simulink model "Moter_Sensor_Integral"  (R2021a)
settings: Solver=FixedStepDiscrete  StartTime=0.0  StopTime=Inf  FixedStep=0.05  RelTol=1e-3
undefined symbols (not defined in the file or in its folder): DiscIntNeverNeededParam
libraries: arduinolib x4, arduinosensorlib x1
settings Model: SimulationMode=external  SILPILModeSetting=veronly  ExtModeTrigDuration=2  Creator=Samsung  LastModifiedBy=Samsung
settings SolverCC: AutoInsertRateTranBlk=on
settings OptimizationCC: EnhancedBackFolding=on  PassReuseOutputArgsAs=Individual arguments  ZeroExternalMemoryAtStartup=off  ZeroInternalMemoryAtStartup=off  MaxStackSize=64  OptimizeBlockOrder=speed  DifferentSizesBufferReuse=on  OptimizationCustomize=off  EfficientTunableParamExpr=on
settings DebuggingCC: ParameterTunabilityLossMsg=error
settings HardwareCC: ProdBitPerPointer=32  ProdBitPerSizeT=32  ProdBitPerPtrDiffT=32  ProdLargestAtomicInteger=Long  ProdLargestAtomicFloat=Double  ProdWordSize=32  ProdHWDeviceType=ARM Compatible->ARM Cortex
settings SFSimCC: MATLABDynamicMemAlloc=off
settings RTWCC: SystemTargetFile=ert.tlc  HardwareBoard=Arduino Nano 33 BLE Sense  TemplateMakefile=ert_default_tmf  Toolchain=Arduino ARM MBED  BuildConfiguration=Faster Runs
settings CodeAppCC: ForceParamTrailComments=on  IgnoreCustomStorageClasses=off  OperatorAnnotations=on  SimulinkDataObjDesc=on  SFDataObjDesc=on  InsertBlockDesc=on
settings ERTTargetCC: SupportContinuousTime=on  SupportVariableSizeSignals=on  ExtMode=on  ExtModeTransport=3  ExtModeStaticAlloc=on  ExtModeStaticAllocSize=65536  ExtModeMexFile=ext_xcp  ExtModeMexArgs=0 16 921600  ExtModeIntrfLevel=Level2 - Open

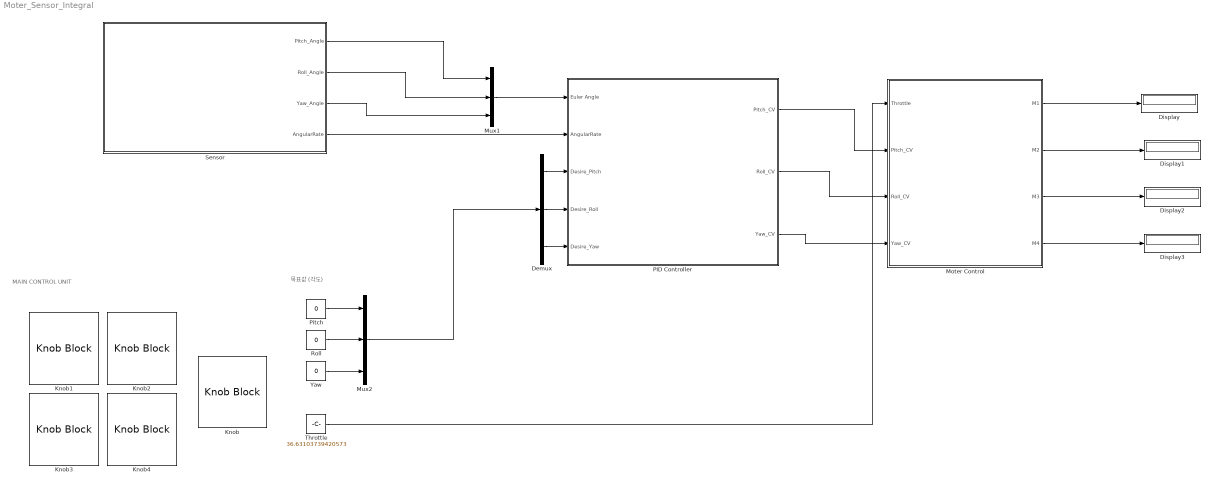
== system Moter_Sensor_Integral ==
  note: MAIN CONTROL UNIT
  note: 목표값 (각도)
  Demux : Demux  Outputs=3
  Display{,1..3} (4 alike) : Display
  Knob : KnobBlock  ScaleMax=200
  Knob1 : KnobBlock  ScaleMax=15
  Knob2 : KnobBlock  ScaleMax=0.1
  Knob3 : KnobBlock  ScaleMin=1  ScaleMax=15
  Knob4 : KnobBlock  ScaleMax=0.1
  Moter Control : Subsystem
  Mux1 : Mux  Inputs=3
  Mux2 : Mux  Inputs=3
  PID Controller : Subsystem
  Pitch : Constant  Value=0
  Roll : Constant  Value=0
  Sensor : Subsystem
  Throttle : Constant  Value=36.63103739420573
  Yaw : Constant  Value=0
  wires:
  PID Controller/1(Pitch_CV) -> Moter Control/2(Pitch_CV)
  PID Controller/2(Roll_CV) -> Moter Control/3(Roll_CV)
  PID Controller/3(Yaw_CV) -> Moter Control/4(Yaw_CV)
  Mux1/1 -> PID Controller/1(Euler Angle)
  Sensor/1(" Pitch_Angle") -> Mux1/1
  Sensor/2(" Roll_Angle") -> Mux1/2
  Sensor/3(Yaw_Angle) -> Mux1/3
  Roll/1 -> Mux2/2
  Pitch/1 -> Mux2/1
  Yaw/1 -> Mux2/3
  Sensor/4(AngularRate) -> PID Controller/2(AngularRate)
  Demux/2 -> PID Controller/4(Desire_Roll)
  Demux/1 -> PID Controller/3(Desire_Pitch)
  Demux/3 -> PID Controller/5(Desire_Yaw)
  Mux2/1 -> Demux/1
  Throttle/1 -> Moter Control/1(Throttle)
  Moter Control/4(M4) -> Display3/1
  Moter Control/3(M3) -> Display2/1
  Moter Control/2(M2) -> Display1/1
  Moter Control/1(M1) -> Display/1

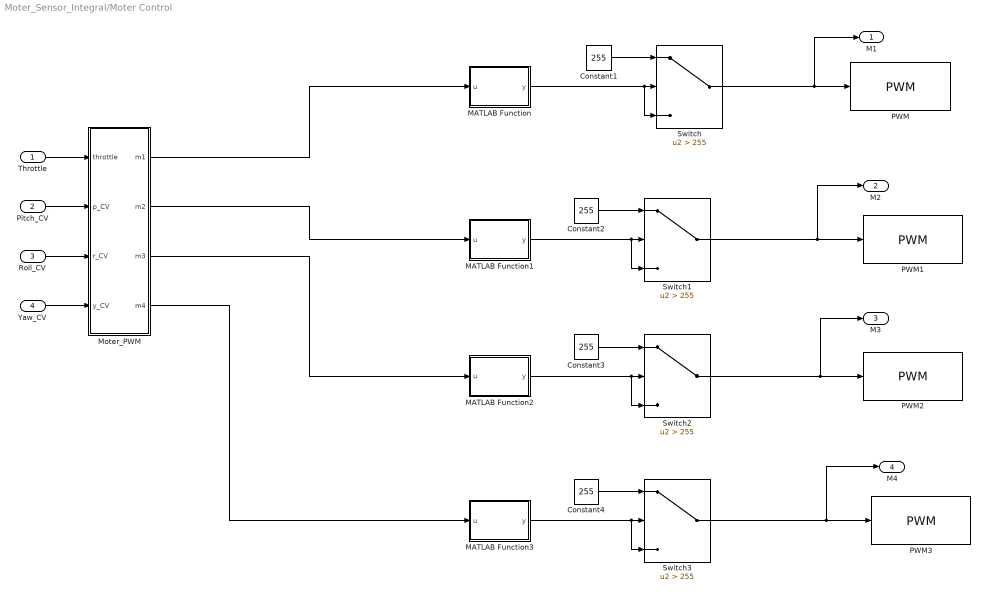
== system Moter_Sensor_Integral/Moter Control ==
  Throttle : Inport
  Pitch_CV : Inport  Port=2
  Roll_CV : Inport  Port=3
  Yaw_CV : Inport  Port=4
  Constant{1..4} (4 alike) : Constant  Value=255
  MATLAB Function : MATLAB Function  TreatAsAtomicUnit=on
  MATLAB Function1 : MATLAB Function  TreatAsAtomicUnit=on
  MATLAB Function2 : MATLAB Function  TreatAsAtomicUnit=on
  MATLAB Function3 : MATLAB Function  TreatAsAtomicUnit=on
  Moter_PWM : MATLAB Function  TreatAsAtomicUnit=on
  PWM : arduinolib/PWM  pinNumber=12  frequencyType=Default  desiredFrequency=490.2  achievableFrequency=490.2
  PWM1 : arduinolib/PWM  pinNumber=8  frequencyType=Default  desiredFrequency=490.2  achievableFrequency=490.2
  PWM2 : arduinolib/PWM  pinNumber=7  frequencyType=Default  desiredFrequency=490.2  achievableFrequency=490.2
  PWM3 : arduinolib/PWM  pinNumber=9  frequencyType=Default  desiredFrequency=490.2  achievableFrequency=490.2
  Switch{,1..3} (4 alike) : Switch  Criteria=u2 > Threshold  Threshold=255
  M1 : Outport
  M2 : Outport  Port=2
  M3 : Outport  Port=3
  M4 : Outport  Port=4
  wires:
  Moter_PWM/1(m1) -> MATLAB Function/1(u)
  Constant1/1 -> Switch/1
  MATLAB Function/1(y) -> Switch/3, Switch/2
  Switch/1 -> M1/1, PWM/1
  Moter_PWM/2(m2) -> MATLAB Function1/1(u)
  Moter_PWM/3(m3) -> MATLAB Function2/1(u)
  Moter_PWM/4(m4) -> MATLAB Function3/1(u)
  MATLAB Function1/1(y) -> Switch1/3, Switch1/2
  Constant2/1 -> Switch1/1
  MATLAB Function2/1(y) -> Switch2/3, Switch2/2
  Constant3/1 -> Switch2/1
  Switch1/1 -> M2/1, PWM1/1
  Switch2/1 -> M3/1, PWM2/1
  MATLAB Function3/1(y) -> Switch3/3, Switch3/2
  Constant4/1 -> Switch3/1
  Switch3/1 -> M4/1, PWM3/1
  Throttle/1 -> Moter_PWM/1(throttle)
  Pitch_CV/1 -> Moter_PWM/2(p_CV)
  Roll_CV/1 -> Moter_PWM/3(r_CV)
  Yaw_CV/1 -> Moter_PWM/4(y_CV)

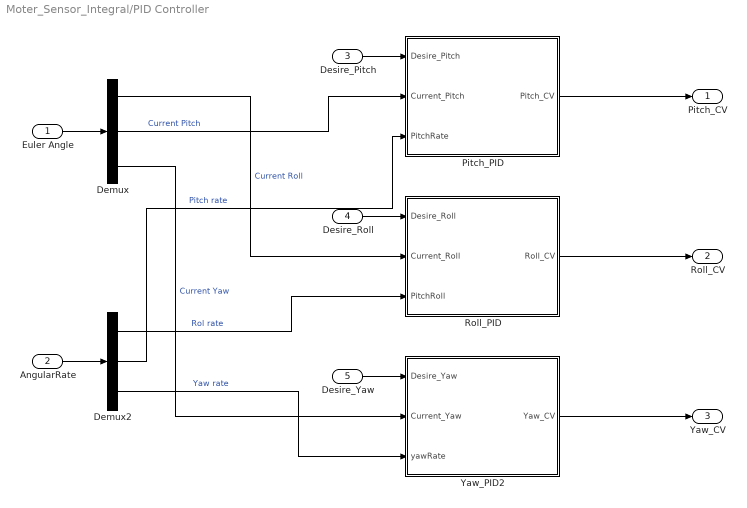
== system Moter_Sensor_Integral/PID Controller ==
  Euler Angle : Inport
  AngularRate : Inport  Port=2
  Desire_Pitch : Inport  Port=3
  Desire_Roll : Inport  Port=4
  Desire_Yaw : Inport  Port=5
  Demux : Demux  Outputs=3
  Demux2 : Demux  Outputs=3
  Pitch_PID : Subsystem
  Roll_PID : Subsystem
  Yaw_PID2 : Subsystem
  Pitch_CV : Outport
  Roll_CV : Outport  Port=2
  Yaw_CV : Outport  Port=3
  wires:
  Euler Angle/1 -> Demux/1
  AngularRate/1 -> Demux2/1
  Desire_Pitch/1 -> Pitch_PID/1(Desire_Pitch)
  Desire_Yaw/1 -> Yaw_PID2/1(Desire_Yaw)
  Demux/3 -> Yaw_PID2/2(Current_Yaw)  "Current Yaw"
  Demux2/3 -> Yaw_PID2/3(yawRate)  "Yaw rate"
  Pitch_PID/1(Pitch_CV) -> Pitch_CV/1
  Roll_PID/1(Roll_CV) -> Roll_CV/1
  Yaw_PID2/1(Yaw_CV) -> Yaw_CV/1
  Desire_Roll/1 -> Roll_PID/1(Desire_Roll)
  Demux/1 -> Roll_PID/2(Current_Roll)  "Current Roll"
  Demux2/1 -> Roll_PID/3(PitchRoll)  "Rol rate"
  Demux/2 -> Pitch_PID/2(Current_Pitch)  "Current Pitch"
  Demux2/2 -> Pitch_PID/3(PitchRate)  "Pitch rate"

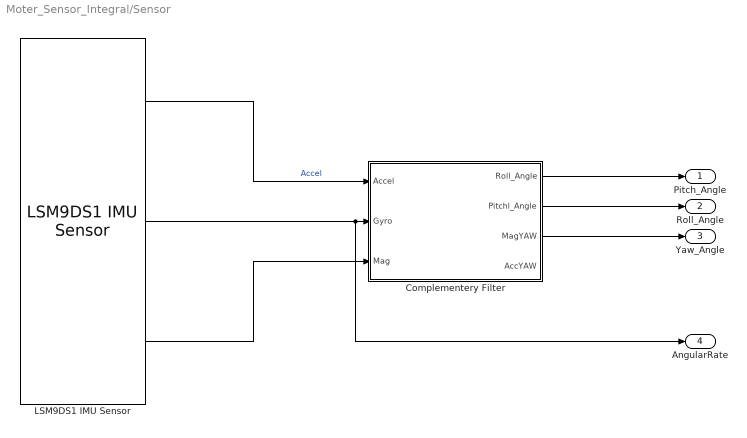
== system Moter_Sensor_Integral/Sensor ==
  Complementery Filter : Subsystem
  LSM9DS1 IMU Sensor : arduinosensorlib/LSM9DS1 IMU Sensor  AccelandGyroAddress=0x6B  MagnetometerAddress=0x1E  EnableAccel=on  EnableGyro=on  EnableMag=on  AccelerometerOutputDataRate=476 Hz  AccelerometerFullScaleRange=+/- 8g  AccelerometerBandwidth=50 Hz  GyroscopeOutputDataRate=119 Hz  GyroscopeFullScaleRange=245 dps  GyroscopeBandwidthMode=0  GyroscopeHighPassFilterEnabled=on  GyroscopeHighPassFilterMode=0  MagnetometerOutputDataRate=40 Hz  MagnetometerFullScaleRange=+/- 4 gauss  SampleTime=0.05
      settings: SourceProductBaseCode=ARDUINO
  " Pitch_Angle" : Outport
  " Roll_Angle" : Outport  Port=2
  Yaw_Angle : Outport  Port=3
  AngularRate : Outport  Port=4
  wires:
  LSM9DS1 IMU Sensor/1 -> Complementery Filter/1(Accel)  "Accel"
  LSM9DS1 IMU Sensor/2 -> AngularRate/1, Complementery Filter/2(Gyro)
  LSM9DS1 IMU Sensor/3 -> Complementery Filter/3(Mag)
  Complementery Filter/1(" Roll_Angle") -> " Pitch_Angle"/1
  Complementery Filter/2(" Pitchl_Angle") -> " Roll_Angle"/1
  Complementery Filter/3(MagYAW) -> Yaw_Angle/1

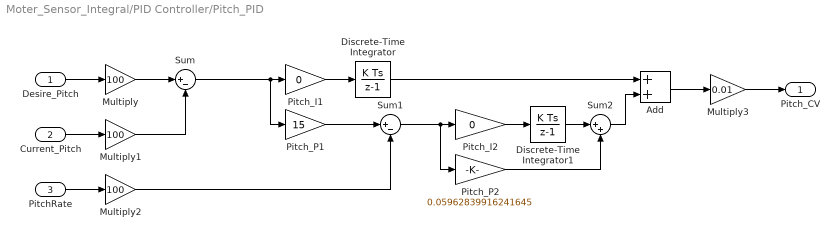
== system Moter_Sensor_Integral/PID Controller/Pitch_PID ==
  Desire_Pitch : Inport
  Current_Pitch : Inport  Port=2
  PitchRate : Inport  Port=3
  Add : Sum
  Discrete-Time Integrator : DiscreteIntegrator  SampleTime=-1  ICPrevOutput=DiscIntNeverNeededParam  ICPrevScaledInput=DiscIntNeverNeededParam
  Discrete-Time Integrator1 : DiscreteIntegrator  SampleTime=-1  ICPrevOutput=DiscIntNeverNeededParam  ICPrevScaledInput=DiscIntNeverNeededParam
  Multiply : Gain  Gain=100
  Multiply1 : Gain  Gain=100
  Multiply2 : Gain  Gain=100
  Multiply3 : Gain  Gain=0.01
  Pitch_I1 : Gain  Gain=0
  Pitch_I2 : Gain  Gain=0
  Pitch_P1 : Gain  Gain=15
  Pitch_P2 : Gain  Gain=0.05962839916241645
  Sum : Sum  Inputs=|+-
  Sum1 : Sum  Inputs=|+-
  Sum2 : Sum  Inputs=|++
  Pitch_CV : Outport
  wires:
  Desire_Pitch/1 -> Multiply/1
  Current_Pitch/1 -> Multiply1/1
  Sum/1 -> Pitch_P1/1, Pitch_I1/1
  Pitch_I1/1 -> Discrete-Time Integrator/1
  Pitch_P1/1 -> Sum1/1
  PitchRate/1 -> Multiply2/1
  Sum1/1 -> Pitch_P2/1, Pitch_I2/1
  Discrete-Time Integrator/1 -> Add/1
  Pitch_I2/1 -> Discrete-Time Integrator1/1
  Pitch_P2/1 -> Sum2/2
  Sum2/1 -> Add/2
  Discrete-Time Integrator1/1 -> Sum2/1
  Multiply/1 -> Sum/1
  Multiply1/1 -> Sum/2
  Multiply2/1 -> Sum1/2
  Add/1 -> Multiply3/1
  Multiply3/1 -> Pitch_CV/1

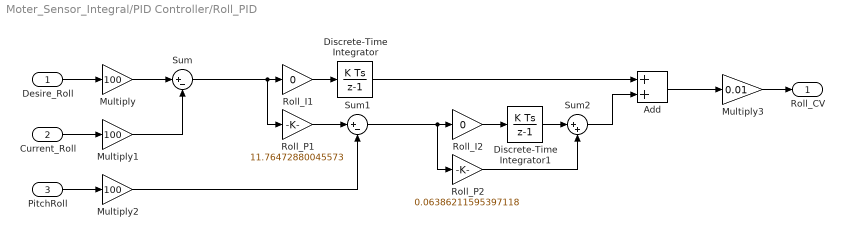
== system Moter_Sensor_Integral/PID Controller/Roll_PID ==
  Desire_Roll : Inport
  Current_Roll : Inport  Port=2
  PitchRoll : Inport  Port=3
  Add : Sum
  Discrete-Time Integrator : DiscreteIntegrator  SampleTime=-1  ICPrevOutput=DiscIntNeverNeededParam  ICPrevScaledInput=DiscIntNeverNeededParam
  Discrete-Time Integrator1 : DiscreteIntegrator  SampleTime=-1  ICPrevOutput=DiscIntNeverNeededParam  ICPrevScaledInput=DiscIntNeverNeededParam
  Multiply : Gain  Gain=100
  Multiply1 : Gain  Gain=100
  Multiply2 : Gain  Gain=100
  Multiply3 : Gain  Gain=0.01
  Roll_I1 : Gain  Gain=0
  Roll_I2 : Gain  Gain=0
  Roll_P1 : Gain  Gain=11.76472880045573
  Roll_P2 : Gain  Gain=0.06386211595397118
  Sum : Sum  Inputs=|+-
  Sum1 : Sum  Inputs=|+-
  Sum2 : Sum  Inputs=|++
  Roll_CV : Outport
  wires:
  Roll_P2/1 -> Sum2/2
  Sum1/1 -> Roll_P2/1, Roll_I2/1
  Roll_I2/1 -> Discrete-Time Integrator1/1
  Discrete-Time Integrator1/1 -> Sum2/1
  Discrete-Time Integrator/1 -> Add/1
  Sum/1 -> Roll_P1/1, Roll_I1/1
  Sum2/1 -> Add/2
  Desire_Roll/1 -> Multiply/1
  PitchRoll/1 -> Multiply2/1
  Roll_P1/1 -> Sum1/1
  Current_Roll/1 -> Multiply1/1
  Roll_I1/1 -> Discrete-Time Integrator/1
  Add/1 -> Multiply3/1
  Multiply/1 -> Sum/1
  Multiply1/1 -> Sum/2
  Multiply2/1 -> Sum1/2
  Multiply3/1 -> Roll_CV/1

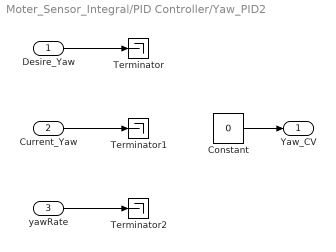
== system Moter_Sensor_Integral/PID Controller/Yaw_PID2 ==
  Desire_Yaw : Inport
  Current_Yaw : Inport  Port=2
  yawRate : Inport  Port=3
  Constant : Constant  Value=0
  Terminator : Terminator
  Terminator1 : Terminator
  Terminator2 : Terminator
  Yaw_CV : Outport
  wires:
  Desire_Yaw/1 -> Terminator/1
  Current_Yaw/1 -> Terminator1/1
  yawRate/1 -> Terminator2/1
  Constant/1 -> Yaw_CV/1

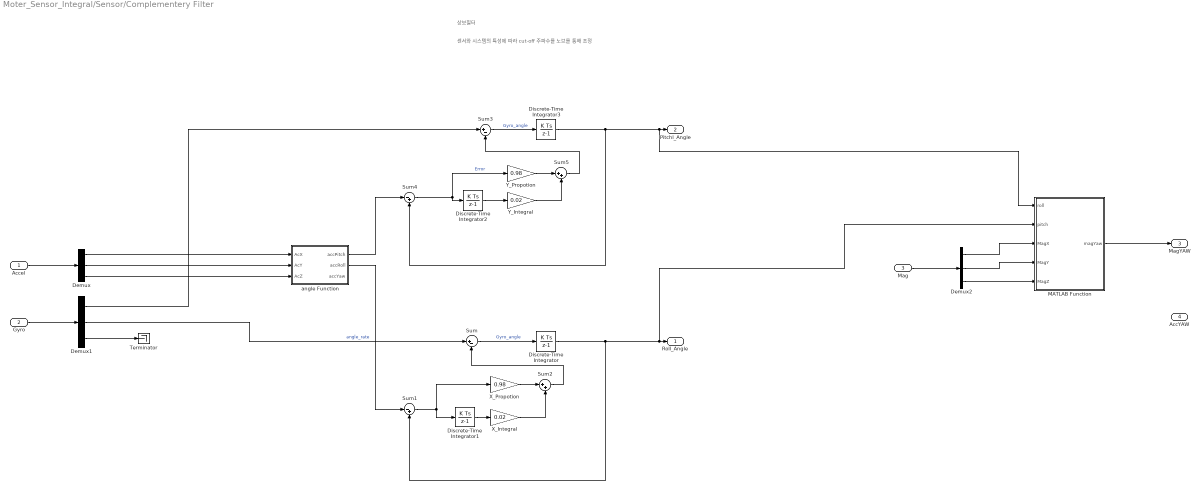
== system Moter_Sensor_Integral/Sensor/Complementery Filter ==
  note: 센서와 시스템의 특성에 따라 cut-off 주파수를 노브를 통해 조정
  note: 상보필터
  Accel : Inport
  Gyro : Inport  Port=2
  Mag : Inport  Port=3
  Demux : Demux  Outputs=3
  Demux1 : Demux  Outputs=3
  Demux2 : Demux  Outputs=3
  Discrete-Time Integrator{,1..3} (4 alike) : DiscreteIntegrator  SampleTime=-1  ICPrevOutput=DiscIntNeverNeededParam  ICPrevScaledInput=DiscIntNeverNeededParam
  MATLAB Function : MATLAB Function  TreatAsAtomicUnit=on
  Sum : Sum  Inputs=|+-
  Sum1 : Sum  Inputs=|-+
  Sum2 : Sum  Inputs=|++
  Sum3 : Sum  Inputs=|+-
  Sum4 : Sum  Inputs=|-+
  Sum5 : Sum  Inputs=|++
  Terminator : Terminator
  X_Integral : Gain  Gain=0.02
  X_Propotion : Gain  Gain=0.98
  Y_Integral : Gain  Gain=0.02
  Y_Propotion : Gain  Gain=0.98
  angle Function : MATLAB Function  TreatAsAtomicUnit=on
  " Roll_Angle" : Outport
  " Pitchl_Angle" : Outport  Port=2
  MagYAW : Outport  Port=3
  " AccYAW" : Outport  Port=4
  wires:
  X_Integral/1 -> Sum2/2
  Sum/1 -> Discrete-Time Integrator/1  "Gyro_angle"
  Discrete-Time Integrator1/1 -> X_Integral/1
  X_Propotion/1 -> Sum2/1
  Sum1/1 -> Discrete-Time Integrator1/1, X_Propotion/1
  Sum2/1 -> Sum/2
  Y_Propotion/1 -> Sum5/1
  Y_Integral/1 -> Sum5/2
  Sum3/1 -> Discrete-Time Integrator3/1  "Gyro_angle"
  Sum5/1 -> Sum3/2
  Sum4/1 -> Discrete-Time Integrator2/1, Y_Propotion/1  "Error"
  Discrete-Time Integrator3/1 -> MATLAB Function/1(roll), " Pitchl_Angle"/1, Sum4/2
  Discrete-Time Integrator/1 -> MATLAB Function/2(pitch), " Roll_Angle"/1, Sum1/2
  Demux/1 -> angle Function/1(AcX)
  Demux/2 -> angle Function/2(AcY)
  Demux/3 -> angle Function/3(AcZ)
  Accel/1 -> Demux/1
  Demux1/3 -> Terminator/1
  Gyro/1 -> Demux1/1
  Discrete-Time Integrator2/1 -> Y_Integral/1
  Mag/1 -> Demux2/1
  Demux2/1 -> MATLAB Function/3(MagX)
  Demux2/2 -> MATLAB Function/4(MagY)
  Demux2/3 -> MATLAB Function/5(MagZ)
  MATLAB Function/1(magYaw) -> MagYAW/1
  Demux1/1 -> Sum3/1
  Demux1/2 -> Sum/1  "angle_rate"
  angle Function/1(accPitch) -> Sum4/1
  angle Function/2(accRoll) -> Sum1/1

== matlab function Moter_Sensor_Integral/Sensor/Complementery Filter/MATLAB Function ==
  data: roll input; magYaw output; pitch input; MagX input; MagY input; MagZ input
function magYaw  = Mag2Yaw(roll, pitch, MagX, MagY, MagZ)

Yh = (MagY * cos(roll)) - (MagZ * sin(roll));
Xh = (MagX * cos(pitch)) + (MagY * sin(pitch)) + (MagZ * cos(roll) * sin(pitch));

magYaw = atan(Yh / Xh) * 180/pi;

== matlab function Moter_Sensor_Integral/Sensor/Complementery Filter/angle Function ==
  data: accPitch output; accRoll output; AcX input; AcY input; AcZ input; accYaw output
function [accPitch, accRoll,accYaw] = fcn(AcX,AcY,AcZ)

accPitch = -atan(AcY / (sqrt(AcX^2 + AcZ^2))) * 180/pi;
accRoll = atan(AcX / (sqrt(AcY^2 + AcZ^2))) * 180/pi;
accYaw = atan(AcY / AcZ) * 180/pi;

end

== matlab function Moter_Sensor_Integral/Moter Control/MATLAB Function ==
  data: u input; y output
function y = IsUnderZero(u)
if u < 0
    u = 0;
end

y = u;

== matlab function Moter_Sensor_Integral/Moter Control/MATLAB Function1 ==
  data: u input; y output
function y = IsUnderZero(u)
if u < 0
    u = 0;
end

    y = u;

== matlab function Moter_Sensor_Integral/Moter Control/MATLAB Function2 ==
  data: u input; y output
function y = IsUnderZero(u)
if u < 0
    u = 0;
end

    y = u;

== matlab function Moter_Sensor_Integral/Moter Control/MATLAB Function3 ==
  data: u input; y output
function y = IsUnderZero(u)
if u < 0
    u = 0;
end

    y = u;

== matlab function Moter_Sensor_Integral/Moter Control/Moter_PWM ==
  data: throttle input; m1 output; p_CV input; r_CV input; y_CV input; m2 output; m3 output; m4 output
function [m1, m2, m3, m4] = MoterPWM(throttle, p_CV, r_CV, y_CV)

if throttle == 0
    m1 = 0;
    m2 = 0;
    m3 = 0;
    m4 = 0;

else
    m2 = throttle + p_CV + r_CV + y_CV;
    m4 = throttle - p_CV + r_CV - y_CV;
    m1 = throttle + p_CV - r_CV - y_CV;
    m3 = throttle - p_CV - r_CV + y_CV;
end
